simulink model "Problem_5_Circuit"  (R2020b)
settings: Solver=VariableStepAuto  StartTime=0.0  StopTime=10  RelTol=1e-3
values from neighbouring files (symbols this model uses):
  C = 1/10*10^-6    (= 1e-07)    [Initial_Condition_Circuit.m]
  q = q+5    (= 6)    [Initial_Condition_Circuit.m]
  R = 10    [Initial_Condition_Circuit.m]
settings Model: Creator=Manoj  LastModifiedBy=Windows 10

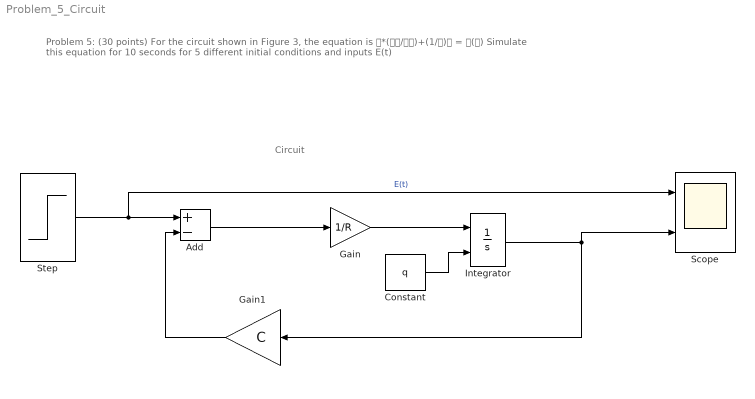
== system Problem_5_Circuit ==
  note: Circuit
  note: Problem 5: (30 points) For the circuit shown in Figure 3, the equation is
      | 𝑅*(𝑑𝑄/𝑑𝑡)+(1/𝐶)𝑄 = 𝐸(𝑡)
      | Simulate this equation for 10 seconds for 5 different initial conditions and inputs E(t)
  Add : Sum  Inputs=+-
  Constant : Constant  Value=q
  Gain : Gain  Gain=1/R
  Gain1 : Gain  Gain=C
  Integrator : Integrator  InitialConditionSource=external
  Scope : Scope  NumInputPorts=2
  Step : Step  SampleTime=0
  wires:
  Step/1 -> Add/1, Scope/1  "E(t)"
  Add/1 -> Gain/1
  Gain1/1 -> Add/2
  Gain/1 -> Integrator/1
  Constant/1 -> Integrator/2
  Integrator/1 -> Scope/2, Gain1/1
